simulink model "Simulation_Model"  (R2024b)
settings: Solver=VariableStepAuto  StartTime=0.0  StopTime=inf  RelTol=1e-3
settings Model: Creator=pc  LastModifiedBy=pc

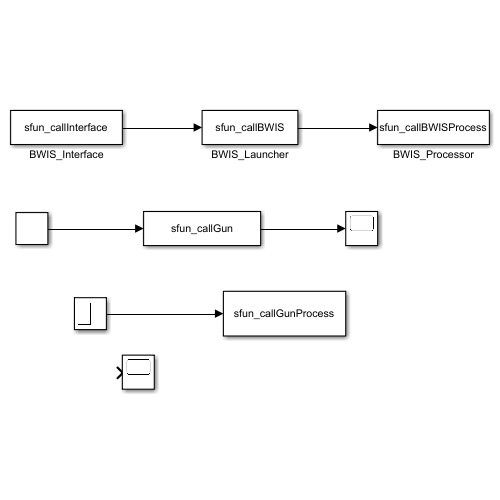
[thumbnail: Simulink's stored preview of the top-level diagram]
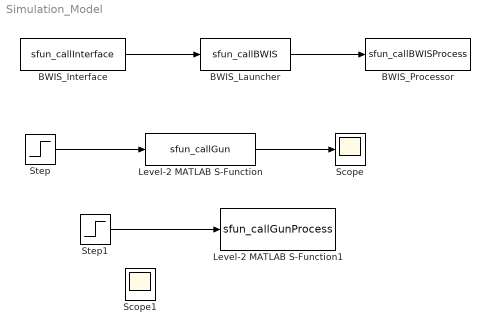
== system Simulation_Model ==
  BWIS_Interface : M-S-Function  FunctionName=sfun_callInterface
      settings: OpenFcn=start_import_gui
  BWIS_Launcher : M-S-Function  FunctionName=sfun_callBWIS  Parameters=paramPath  mask{paramPath=C:\Users\pc\Desktop\BWIS_互作用-helix-非线性特征仿真实例\注波互作用1\指定输入}
      mask prompts: paramPath "求解器路径"
      mask DialogControl ParameterGroupVar Prompt: 参数
  BWIS_Processor : M-S-Function  FunctionName=sfun_callBWISProcess  Parameters=dataDir  mask{dataDir=C:\Users\pc\Desktop\BWIS_互作用-helix-非线性特征仿真实例\注波互作用1\指定输入}
      mask prompts: dataDir "求解器数据路径"
      mask DialogControl ParameterGroupVar Prompt: 参数
  Level-2 MATLAB S-Function : M-S-Function  FunctionName=sfun_callGun
  Level-2 MATLAB S-Function1 : M-S-Function  FunctionName=sfun_callGunProcess
  Scope : Scope
  Scope1 : Scope
  Step : Step  SampleTime=0
  Step1 : Step  Before=1  After=2  SampleTime=0
  wires:
  BWIS_Launcher/1 -> BWIS_Processor/1
  BWIS_Interface/1 -> BWIS_Launcher/1
  Step/1 -> Level-2 MATLAB S-Function/1
  Level-2 MATLAB S-Function/1 -> Scope/1
  Step1/1 -> Level-2 MATLAB S-Function1/1
